simulink model "Irradiancia"  (R2023b)
settings: Solver=VariableStepAuto  StartTime=0.0  StopTime=60  RelTol=1e-8
undefined symbols (not defined in the file or in its folder): sigbuilder_block
settings Model: Creator=Guillermo  LastModifiedBy=Guillermo
settings SolverCC: ZeroCrossAlgorithm=Adaptive
settings DebuggingCC: UnconnectedInputMsg=warning  UnconnectedOutputMsg=warning  UnconnectedLineMsg=warning
settings ModelReferenceCC: EnableRefExpFcnMdlSchedulingChecks=on
settings RTWCC: DLArmComputeVersion=19.05

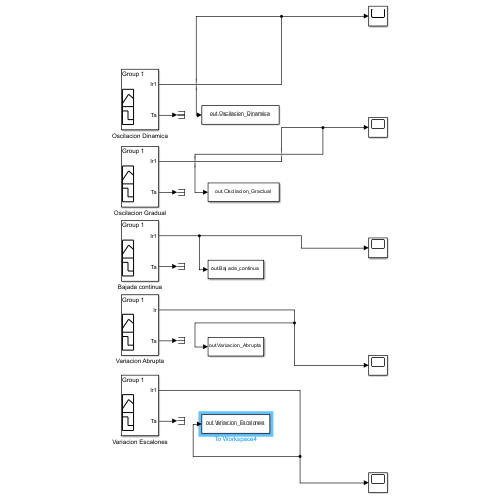
[thumbnail: Simulink's stored preview of the top-level diagram]
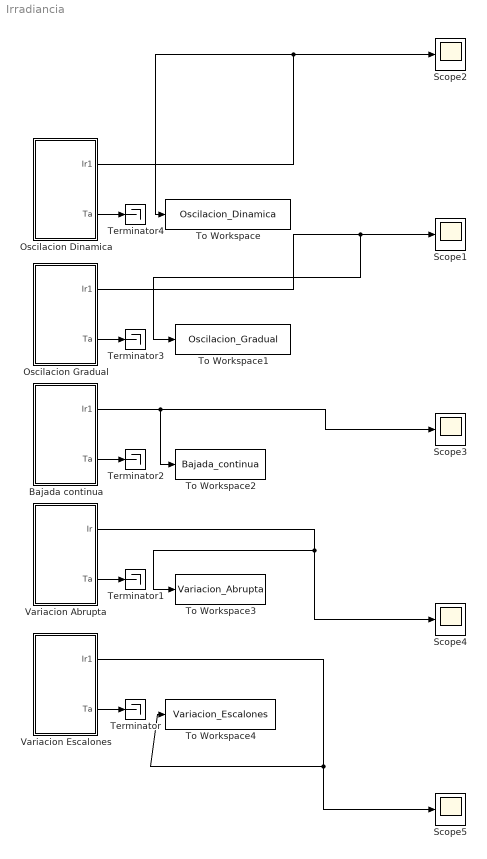
== system Irradiancia ==
  Bajada continua : Subsystem  Tag=STV Subsys  LoadFcn=sigbuilder_block('load');  StartFcn=sigbuilder_block('start');  StopFcn=sigbuilder_block('stop');  ClipboardFcn=sigbuilder_block('clipboard');  mask(Sigbuilder block){tuvar=[0:10]}
      mask help: Simulink:masks:SigbuilderBlock_MD
      mask init:
      | if ~strcmp(get_param(bdroot(gcbh),'SimulationStatus'),'stopped') tuvar = sigbuilder_block('maskInit'); end
      settings: CopyFcn=sigbuilder_block('copy');  DeleteFcn=sigbuilder_block('delete');  ModelCloseFcn=sigbuilder_block('modelClose');  PreSaveFcn=sigbuilder_block('preSave');  PauseFcn=sigbuilder_block('pause');  ContinueFcn=sigbuilder_block('continue');  NameChangeFcn=sigbuilder_block('namechange');  OpenFcn=sigbuilder_block('open',[6 6 1012.5 506.25 ]);  CloseFcn=sigbuilder_block('close');
      mask Display: plot(0, 0, 100, 100,[2, 2, 32, 32, 2], [68, 8, 8, 68, 68],[32, 2], [38, 38], [32, 19, 2],[53, 60, 44], [32, 17, 17, 2],[16, 16, 31, 31]);txt = getActiveGroup(gcbh);text(2, 100, txt,'verticalAlignment', 'top');
  Oscilacion Dinamica : Subsystem  Tag=STV Subsys  LoadFcn=sigbuilder_block('load');  StartFcn=sigbuilder_block('start');  StopFcn=sigbuilder_block('stop');  ClipboardFcn=sigbuilder_block('clipboard');  mask(Sigbuilder block){tuvar=[0:10]}
      mask help: Simulink:masks:SigbuilderBlock_MD
      mask init:
      | if ~strcmp(get_param(bdroot(gcbh),'SimulationStatus'),'stopped') tuvar = sigbuilder_block('maskInit'); end
      settings: CopyFcn=sigbuilder_block('copy');  DeleteFcn=sigbuilder_block('delete');  ModelCloseFcn=sigbuilder_block('modelClose');  PreSaveFcn=sigbuilder_block('preSave');  PauseFcn=sigbuilder_block('pause');  ContinueFcn=sigbuilder_block('continue');  NameChangeFcn=sigbuilder_block('namechange');  OpenFcn=sigbuilder_block('open',[12.75 -266.25 1012.5 506.25 ]);  CloseFcn=sigbuilder_block('close');
      mask Display: plot(0, 0, 100, 100,[2, 2, 32, 32, 2], [68, 8, 8, 68, 68],[32, 2], [38, 38], [32, 19, 2],[53, 60, 44], [32, 17, 17, 2],[16, 16, 31, 31]);txt = getActiveGroup(gcbh);text(2, 100, txt,'verticalAlignment', 'top');
  Oscilacion Gradual : Subsystem  Tag=STV Subsys  LoadFcn=sigbuilder_block('load');  StartFcn=sigbuilder_block('start');  StopFcn=sigbuilder_block('stop');  ClipboardFcn=sigbuilder_block('clipboard');  mask(Sigbuilder block){tuvar=[0:10]}
      mask help: Simulink:masks:SigbuilderBlock_MD
      mask init:
      | if ~strcmp(get_param(bdroot(gcbh),'SimulationStatus'),'stopped') tuvar = sigbuilder_block('maskInit'); end
      settings: CopyFcn=sigbuilder_block('copy');  DeleteFcn=sigbuilder_block('delete');  ModelCloseFcn=sigbuilder_block('modelClose');  PreSaveFcn=sigbuilder_block('preSave');  PauseFcn=sigbuilder_block('pause');  ContinueFcn=sigbuilder_block('continue');  NameChangeFcn=sigbuilder_block('namechange');  OpenFcn=sigbuilder_block('open',[4.5 30.75 1019.25 481.5 ]);  CloseFcn=sigbuilder_block('close');
      mask Display: plot(0, 0, 100, 100,[2, 2, 32, 32, 2], [68, 8, 8, 68, 68],[32, 2], [38, 38], [32, 19, 2],[53, 60, 44], [32, 17, 17, 2],[16, 16, 31, 31]);txt = getActiveGroup(gcbh);text(2, 100, txt,'verticalAlignment', 'top');
  Scope{1..5} (5 alike) : Scope
  Terminator{,1..4} (5 alike) : Terminator
  To Workspace : ToWorkspace  VariableName=Oscilacion_Dinamica  SampleTime=1e-3
  To Workspace1 : ToWorkspace  VariableName=Oscilacion_Gradual  SampleTime=1e-3
  To Workspace2 : ToWorkspace  VariableName=Bajada_continua  SampleTime=1e-3
  To Workspace3 : ToWorkspace  VariableName=Variacion_Abrupta  SampleTime=1e-3
  To Workspace4 : ToWorkspace  VariableName=Variacion_Escalones  SampleTime=1e-3
  Variacion Abrupta : Subsystem  Tag=STV Subsys  LoadFcn=sigbuilder_block('load');  StartFcn=sigbuilder_block('start');  StopFcn=sigbuilder_block('stop');  ClipboardFcn=sigbuilder_block('clipboard');  mask(Sigbuilder block){tuvar=[0:10]}
      mask help: Simulink:masks:SigbuilderBlock_MD
      mask init:
      | if ~strcmp(get_param(bdroot(gcbh),'SimulationStatus'),'stopped') tuvar = sigbuilder_block('maskInit'); end
      settings: CopyFcn=sigbuilder_block('copy');  DeleteFcn=sigbuilder_block('delete');  ModelCloseFcn=sigbuilder_block('modelClose');  PreSaveFcn=sigbuilder_block('preSave');  PauseFcn=sigbuilder_block('pause');  ContinueFcn=sigbuilder_block('continue');  NameChangeFcn=sigbuilder_block('namechange');  OpenFcn=sigbuilder_block('open',[6 6 1012.5 506.25 ]);  CloseFcn=sigbuilder_block('close');
      mask Display: plot(0, 0, 100, 100,[2, 2, 32, 32, 2], [68, 8, 8, 68, 68],[32, 2], [38, 38], [32, 19, 2],[53, 60, 44], [32, 17, 17, 2],[16, 16, 31, 31]);txt = getActiveGroup(gcbh);text(2, 100, txt,'verticalAlignment', 'top');
  Variacion Escalones : Subsystem  Tag=STV Subsys  LoadFcn=sigbuilder_block('load');  StartFcn=sigbuilder_block('start');  StopFcn=sigbuilder_block('stop');  ClipboardFcn=sigbuilder_block('clipboard');  mask(Sigbuilder block){tuvar=[0:10]}
      mask help: Simulink:masks:SigbuilderBlock_MD
      mask init:
      | if ~strcmp(get_param(bdroot(gcbh),'SimulationStatus'),'stopped') tuvar = sigbuilder_block('maskInit'); end
      settings: CopyFcn=sigbuilder_block('copy');  DeleteFcn=sigbuilder_block('delete');  ModelCloseFcn=sigbuilder_block('modelClose');  PreSaveFcn=sigbuilder_block('preSave');  PauseFcn=sigbuilder_block('pause');  ContinueFcn=sigbuilder_block('continue');  NameChangeFcn=sigbuilder_block('namechange');  OpenFcn=sigbuilder_block('open',[6 6 1012.5 506.25 ]);  CloseFcn=sigbuilder_block('close');
      mask Display: plot(0, 0, 100, 100,[2, 2, 32, 32, 2], [68, 8, 8, 68, 68],[32, 2], [38, 38], [32, 19, 2],[53, 60, 44], [32, 17, 17, 2],[16, 16, 31, 31]);txt = getActiveGroup(gcbh);text(2, 100, txt,'verticalAlignment', 'top');
  wires:
  Oscilacion Dinamica/1(Ir1) -> Scope2/1, To Workspace/1
  Oscilacion Gradual/1(Ir1) -> To Workspace1/1, Scope1/1
  Bajada continua/1(Ir1) -> Scope3/1, To Workspace2/1
  Variacion Abrupta/1(Ir) -> Scope4/1, To Workspace3/1
  Variacion Escalones/1(Ir1) -> Scope5/1, To Workspace4/1
  Variacion Escalones/2(Ta) -> Terminator/1
  Variacion Abrupta/2(Ta) -> Terminator1/1
  Bajada continua/2(Ta) -> Terminator2/1
  Oscilacion Gradual/2(Ta) -> Terminator3/1
  Oscilacion Dinamica/2(Ta) -> Terminator4/1

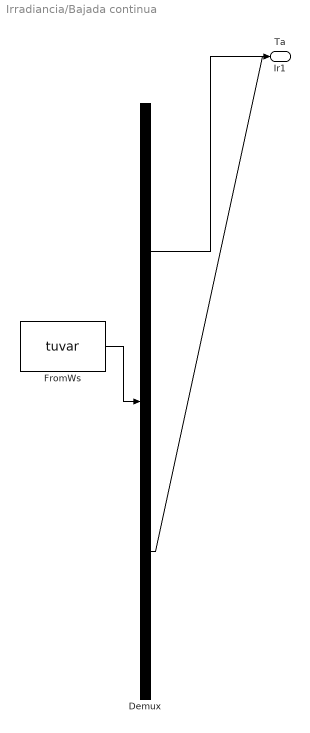
== system Irradiancia/Bajada continua ==
  Demux : Demux  Tag=STV Demux  Outputs=2
      settings: DisplayOption=none
  FromWs : FromWorkspace  Tag=STV FromWs  VariableName=tuvar
      SigBuilderData=|
      | common.afterFinalStr = 'Extrapolate'
      | common.sampleTime = 0
      | dataSet.timeRange = [0 60]
      | dataSet.name = 'Group 1'
      | sbobj.Groups.Name = 'Group 1'
      | sbobj.Groups.Signals(1).Name = 'Ir1'
      | sbobj.Groups.Signals(1).XData = [0 60]
      | sbobj.Groups.Signals(1).YData = [1000 0]
      | sbobj.Groups.Signals(2).Name = 'Ta'
      | sbobj.Groups.Signals(2).XData = [0 60]
      | sbobj.Groups.Signals(2).YData = [22.6 22.6]
      | sbobj.Groups.TimeRange = [0 60]
  Ir1 : Outport  Tag=STV Outport
  Ta : Outport  Tag=STV Outport  Port=2
  wires:
  FromWs/1 -> Demux/1
  Demux/1 -> Ir1/1
  Demux/2 -> Ta/1

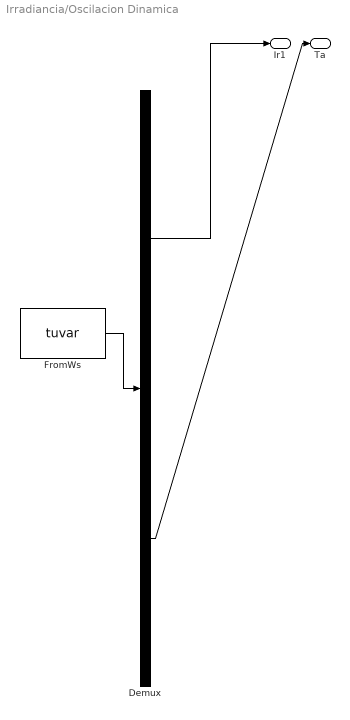
== system Irradiancia/Oscilacion Dinamica ==
  Demux : Demux  Tag=STV Demux  Outputs=2
      settings: DisplayOption=none
  FromWs : FromWorkspace  Tag=STV FromWs  VariableName=tuvar
      SigBuilderData=|
      | common.afterFinalStr = 'Extrapolate'
      | common.sampleTime = 0
      | dataSet.timeRange = [0 60]
      | dataSet.name = 'Group 1'
      | sbobj.Groups.Name = 'Group 1'
      | sbobj.Groups.Signals(1).Name = 'Ir1'
      | sbobj.Groups.Signals(1).XData = [0 1 1.4 7 7.25 10 10.25 10.5 12 12.25 16 16.25 16.5 16.75 18.95 19.5 20 21.05 24 24.5 25 25.25 25.75 29 32 32.25 34 34.25 34.5 34.75 35 37 37.25 41 41.25 41.5 41.75 42 45 45.25 48 48.25 50 50.25 53.75 54 54.25 57 57.25 60]
      | sbobj.Groups.Signals(1).YData = [910 500 295 295 910 910 295 295 295 910 910 295 910 295 295 910 295 910 910 290 910 295 910 910 910 295 295 910 295 910 295 295 910 910 295 910 295 910 910 295 295 910 910 295 295 910 295 295 790 790]
      | sbobj.Groups.Signals(2).Name = 'Ta'
      | sbobj.Groups.Signals(2).XData = [0 60]
      | sbobj.Groups.Signals(2).YData = [22.6 22.6]
      | sbobj.Groups.TimeRange = [0 60]
  Ir1 : Outport  Tag=STV Outport
  Ta : Outport  Tag=STV Outport  Port=2
  wires:
  FromWs/1 -> Demux/1
  Demux/1 -> Ir1/1
  Demux/2 -> Ta/1

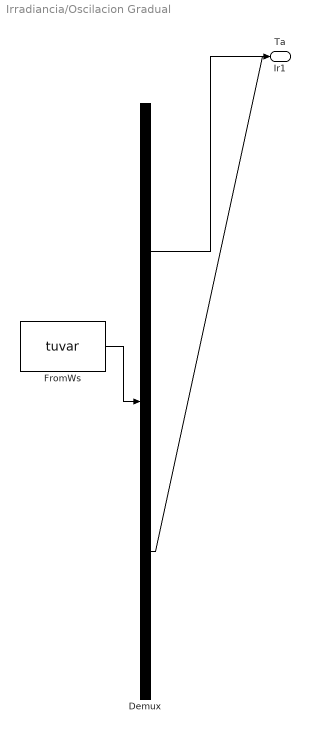
== system Irradiancia/Oscilacion Gradual ==
  Demux : Demux  Tag=STV Demux  Outputs=2
      settings: DisplayOption=none
  FromWs : FromWorkspace  Tag=STV FromWs  VariableName=tuvar
      SigBuilderData=|
      | common.afterFinalStr = 'Extrapolate'
      | common.sampleTime = 0
      | dataSet.timeRange = [0 60]
      | dataSet.name = 'Group 1'
      | sbobj.Groups.Name = 'Group 1'
      | sbobj.Groups.Signals(1).Name = 'Ir1'
      | sbobj.Groups.Signals(1).XData = [0 1 1.4 7 7.25 16.5 16.75 25.25 25.75 34.75 35 37 37.25 45 45.25 48 48.25 50 50.25 57 57.25 57.25 60]
      | sbobj.Groups.Signals(1).YData = [910 500 295 295 910 910 295 295 910 910 295 295 910 910 295 295 910 910 295 295 775 800 800]
      | sbobj.Groups.Signals(2).Name = 'Ta'
      | sbobj.Groups.Signals(2).XData = [0 60]
      | sbobj.Groups.Signals(2).YData = [22.6 22.6]
      | sbobj.Groups.TimeRange = [0 60]
  Ir1 : Outport  Tag=STV Outport
  Ta : Outport  Tag=STV Outport  Port=2
  wires:
  FromWs/1 -> Demux/1
  Demux/1 -> Ir1/1
  Demux/2 -> Ta/1

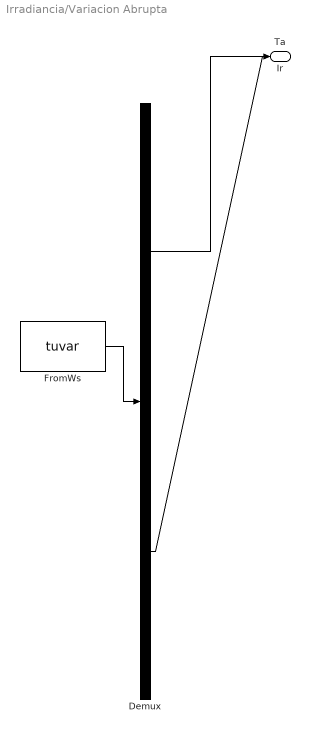
== system Irradiancia/Variacion Abrupta ==
  Demux : Demux  Tag=STV Demux  Outputs=2
      settings: DisplayOption=none
  FromWs : FromWorkspace  Tag=STV FromWs  VariableName=tuvar
      SigBuilderData=|
      | common.afterFinalStr = 'Extrapolate'
      | common.sampleTime = 0
      | dataSet.timeRange = [0 60]
      | dataSet.name = 'Group 1'
      | sbobj.Groups.Name = 'Group 1'
      | sbobj.Groups.Signals(1).Name = 'Ir'
      | sbobj.Groups.Signals(1).XData = [0 20 20.1 40 40.1 60]
      | sbobj.Groups.Signals(1).YData = [800 800 100 100 600 600]
      | sbobj.Groups.Signals(2).Name = 'Ta'
      | sbobj.Groups.Signals(2).XData = [0 60]
      | sbobj.Groups.Signals(2).YData = [22.6 22.6]
      | sbobj.Groups.TimeRange = [0 60]
  Ir : Outport  Tag=STV Outport
  Ta : Outport  Tag=STV Outport  Port=2
  wires:
  FromWs/1 -> Demux/1
  Demux/1 -> Ir/1
  Demux/2 -> Ta/1

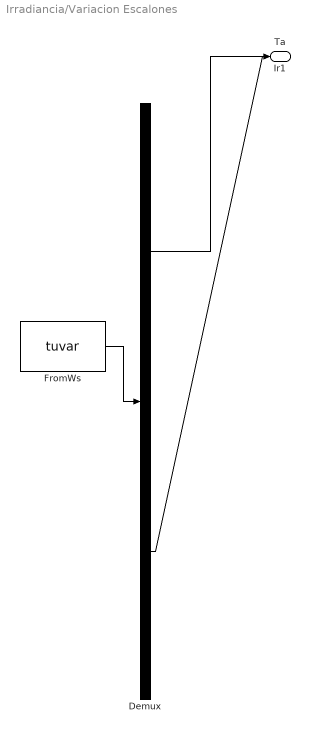
== system Irradiancia/Variacion Escalones ==
  Demux : Demux  Tag=STV Demux  Outputs=2
      settings: DisplayOption=none
  FromWs : FromWorkspace  Tag=STV FromWs  VariableName=tuvar
      SigBuilderData=|
      | common.afterFinalStr = 'Extrapolate'
      | common.sampleTime = 0
      | dataSet.timeRange = [0 60]
      | dataSet.name = 'Group 1'
      | sbobj.Groups.Name = 'Group 1'
      | sbobj.Groups.Signals(1).Name = 'Ir1'
      | sbobj.Groups.Signals(1).XData = [0 15 15.1 30 30.1 45 45.1 60]
      | sbobj.Groups.Signals(1).YData = [1200 1200 900 900 600 600 300 300]
      | sbobj.Groups.Signals(2).Name = 'Ta'
      | sbobj.Groups.Signals(2).XData = [0 60]
      | sbobj.Groups.Signals(2).YData = [22.6 22.6]
      | sbobj.Groups.TimeRange = [0 60]
  Ir1 : Outport  Tag=STV Outport
  Ta : Outport  Tag=STV Outport  Port=2
  wires:
  FromWs/1 -> Demux/1
  Demux/1 -> Ir1/1
  Demux/2 -> Ta/1
